simulink model "drive"  (R2024b)
settings: Solver=VariableStepAuto  StartTime=0.0  StopTime=10.0  RelTol=1e-3
InitFcn:
  | driveIni
values from neighbouring files (symbols this model uses):
  Par = problMatrices(Par)    [driveIni.m]
  psiR0 = [0.91; 0]    [driveIni.m]
  psiS0 = [1; 0]    [driveIni.m]
settings Model: Creator=PetrosK  LastModifiedBy=horak
settings DebuggingCC: UnderspecifiedInitializationDetection=Classic  MergeDetectMultiDrivingBlocksExec=none
settings ModelReferenceCC: PropagateSignalLabelsOutOfModel=off

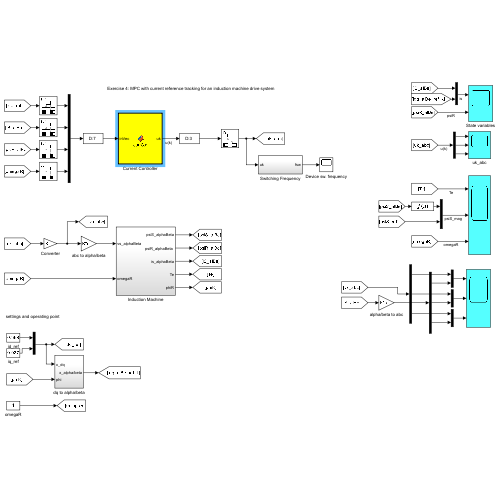
[thumbnail: Simulink's stored preview of the top-level diagram]
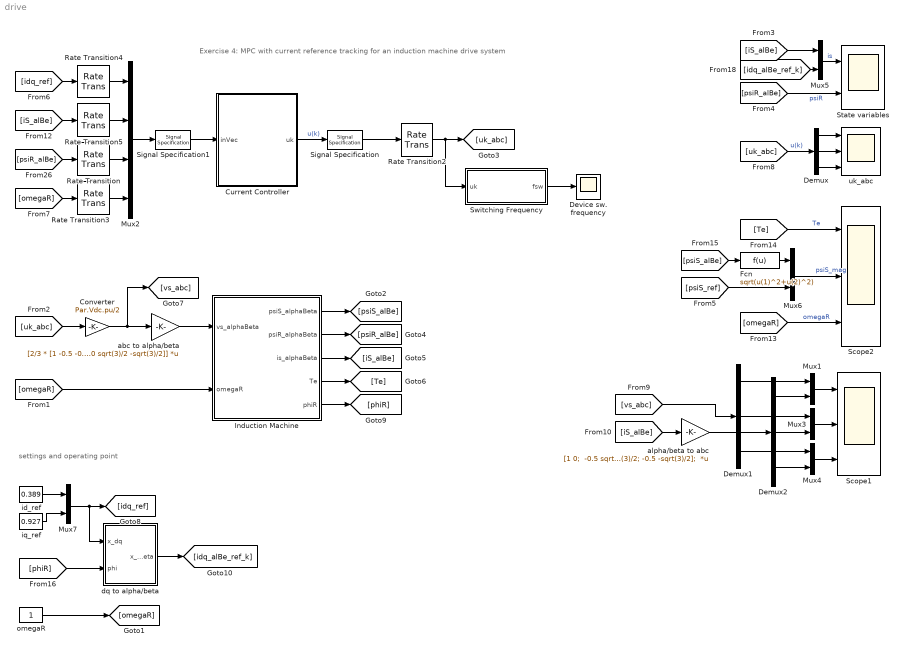
== system drive ==
  note: settings and operating point
  note: Exercise 4: MPC with current reference tracking for an induction machine drive system
  Converter : Gain  Gain=Par.Vdc.pu/2  SaturateOnIntegerOverflow=on  OutDataTypeStr=Inherit: Same as input  ParamDataTypeStr=Inherit: Same as input
  Current Controller : MATLAB Function  TreatAsAtomicUnit=on
  Demux : Demux  Outputs=3
  Demux1 : Demux  Outputs=3
  Demux2 : Demux  Outputs=3
  Device sw. frequency : Scope
  Fcn : Fcn  Expr=sqrt(u(1)^2+u(2)^2)
  Induction Machine : Subsystem
  Mux{1,3..7} (6 alike) : Mux  Inputs=2
  Mux2 : Mux
  Rate Transition{,3..5} (4 alike) : RateTransition  Deterministic=off  OutPortSampleTime=Par.Ts.control
  Rate Transition2 : RateTransition  OutPortSampleTime=Par.Ts.system
  Scope1 : Scope  NumInputPorts=3
  Scope2 : Scope  NumInputPorts=3
  Signal Specification : SignalSpecification  Dimensions=3
  Signal Specification1 : SignalSpecification  Dimensions=7
  State variables : Scope  NumInputPorts=2
  Switching Frequency : Subsystem
  abc to alpha/beta : Gain  Gain=[2/3 * [1 -0.5 -0.5;0 sqrt(3)/2 -sqrt(3)/2]]  Multiplication=Matrix(K*u)  SaturateOnIntegerOverflow=on  OutDataTypeStr=Inherit: Same as input  ParamDataTypeStr=Inherit: Same as input
  alpha/beta to abc : Gain  Gain="[1 0;  -0.5 sqrt(3)/2; -0.5 -sqrt(3)/2];"  Multiplication=Matrix(K*u)  SaturateOnIntegerOverflow=on  OutDataTypeStr=Inherit: Same as input  ParamDataTypeStr=Inherit: Same as input
  dq to alpha/beta : Subsystem
  id_ref : Constant  Value=0.389
  iq_ref : Constant  Value=0.927
  omegaR : Constant
  uk_abc : Scope  NumInputPorts=3
  wires:
  abc to alpha/beta/1 -> Induction Machine/1(vs_alphaBeta)
  [omegaR] -> Induction Machine/2(omegaR)
  [psiR_alBe] -> Rate Transition/1
  Current Controller/1(uk) -> Signal Specification/1  "u(k)"
  [omegaR] -> Rate Transition3/1
  Mux2/1 -> Signal Specification1/1
  Rate Transition3/1 -> Mux2/4
  Rate Transition/1 -> Mux2/3
  Signal Specification/1 -> Rate Transition2/1
  Rate Transition2/1 -> Switching Frequency/1(uk), [uk_abc]
  Signal Specification1/1 -> Current Controller/1(inVec)
  [uk_abc] -> Converter/1
  Converter/1 -> [vs_abc], abc to alpha/beta/1
  [psiR_alBe] -> State variables/2  "psiR"
  [uk_abc] -> Demux/1  "u(k)"
  Demux/1 -> uk_abc/1
  Demux/2 -> uk_abc/2
  Demux/3 -> uk_abc/3
  Induction Machine/1(psiS_alphaBeta) -> [psiS_alBe]
  Induction Machine/2("psiR_alphaBeta ") -> [psiR_alBe]
  Induction Machine/3(is_alphaBeta) -> [iS_alBe]
  Induction Machine/4(Te) -> [Te]
  Mux1/1 -> Scope1/1
  Mux3/1 -> Scope1/2
  Mux4/1 -> Scope1/3
  Demux1/1 -> Mux1/1
  alpha/beta to abc/1 -> Demux2/1
  Demux2/1 -> Mux1/2
  [iS_alBe] -> alpha/beta to abc/1
  Demux1/2 -> Mux3/1
  Demux1/3 -> Mux4/1
  Demux2/2 -> Mux3/2
  Demux2/3 -> Mux4/2
  [vs_abc] -> Demux1/1
  [omegaR] -> Scope2/3  "omegaR"
  Mux6/1 -> Scope2/2  "psiS_mag"
  [psiS_alBe] -> Fcn/1
  Rate Transition5/1 -> Mux2/2
  Rate Transition4/1 -> Mux2/1
  Fcn/1 -> Mux6/1
  [psiS_ref] -> Mux6/2
  omegaR/1 -> [omegaR]
  Switching Frequency/1(fsw) -> Device sw. frequency/1
  [idq_ref] -> Rate Transition4/1
  [iS_alBe] -> Rate Transition5/1
  [Te] -> Scope2/1  "Te"
  Mux7/1 -> dq to alpha/beta/1(x_dq), [idq_ref]
  [phiR] -> dq to alpha/beta/2(phi)
  Induction Machine/5(phiR) -> [phiR]
  dq to alpha/beta/1(x_alpha/beta) -> [idq_alBe_ref_k]
  Mux5/1 -> State variables/1  "is"
  [iS_alBe] -> Mux5/1
  [idq_alBe_ref_k] -> Mux5/2
  id_ref/1 -> Mux7/1
  iq_ref/1 -> Mux7/2

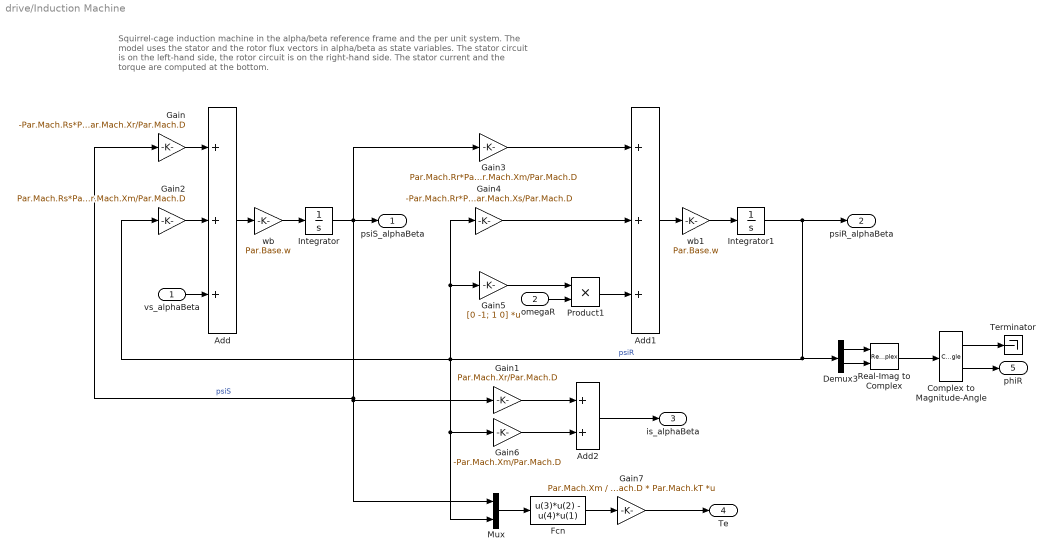
== system drive/Induction Machine ==
  note: Squirrel-cage induction machine in the alpha/beta reference frame and the per unit system.
      | The model uses the stator and the rotor flux vectors in alpha/beta as state variables.
      | The stator circuit is on the left-hand side, the rotor circuit is on the right-hand side.
      | The stator current and the torque are computed at the bottom.
  vs_alphaBeta : Inport
  omegaR : Inport  Port=2
  Add : Sum  Inputs=+++
  Add1 : Sum  Inputs=+++
  Add2 : Sum
  Complex to Magnitude-Angle : ComplexToMagnitudeAngle
  Demux3 : Demux  Outputs=2
  Fcn : Fcn  Expr=u(3)*u(2) - u(4)*u(1)
  Gain : Gain  Gain=-Par.Mach.Rs*Par.Mach.Xr/Par.Mach.D
  Gain1 : Gain  Gain=Par.Mach.Xr/Par.Mach.D
  Gain2 : Gain  Gain=Par.Mach.Rs*Par.Mach.Xm/Par.Mach.D
  Gain3 : Gain  Gain=Par.Mach.Rr*Par.Mach.Xm/Par.Mach.D
  Gain4 : Gain  Gain=-Par.Mach.Rr*Par.Mach.Xs/Par.Mach.D
  Gain5 : Gain  Gain=[0 -1; 1 0]  Multiplication=Matrix(K*u)
  Gain6 : Gain  Gain=-Par.Mach.Xm/Par.Mach.D
  Gain7 : Gain  Gain=Par.Mach.Xm / Par.Mach.D * Par.Mach.kT  Multiplication=Matrix(K*u)
  Integrator : Integrator  InitialCondition=psiS0
  Integrator1 : Integrator  InitialCondition=psiR0
  Mux : Mux  Inputs=2
  Product1 : Product
  Real-Imag to Complex : RealImagToComplex
  Terminator : Terminator
  wb : Gain  Gain=Par.Base.w
  wb1 : Gain  Gain=Par.Base.w
  psiS_alphaBeta : Outport
  "psiR_alphaBeta " : Outport  Port=2
  is_alphaBeta : Outport  Port=3
  Te : Outport  Port=4
  phiR : Outport  Port=5
  wires:
  vs_alphaBeta/1 -> Add/3
  Gain/1 -> Add/1
  Add/1 -> wb/1
  Gain3/1 -> Add1/1
  Add1/1 -> wb1/1
  Gain4/1 -> Add1/2
  Product1/1 -> Add1/3
  Gain2/1 -> Add/2
  Integrator/1 -> Gain3/1, psiS_alphaBeta/1, Mux/1, Gain1/1, Gain/1  "psiS"
  Integrator1/1 -> Demux3/1, Gain2/1, Mux/2, Gain6/1, Gain4/1, Gain5/1, "psiR_alphaBeta "/1  "psiR"
  Gain1/1 -> Add2/1
  Gain6/1 -> Add2/2
  Add2/1 -> is_alphaBeta/1
  Fcn/1 -> Gain7/1
  Gain7/1 -> Te/1
  Gain5/1 -> Product1/1
  omegaR/1 -> Product1/2
  Mux/1 -> Fcn/1
  wb1/1 -> Integrator1/1
  wb/1 -> Integrator/1
  Demux3/1 -> Real-Imag to Complex/1
  Demux3/2 -> Real-Imag to Complex/2
  Real-Imag to Complex/1 -> Complex to Magnitude-Angle/1
  Complex to Magnitude-Angle/2 -> phiR/1
  Complex to Magnitude-Angle/1 -> Terminator/1

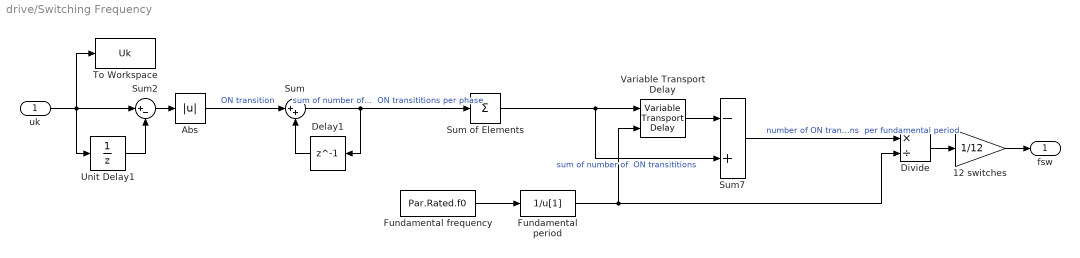
== system drive/Switching Frequency ==
  uk : Inport
  12 switches : Gain  Gain=1/12
  Abs : Abs  SaturateOnIntegerOverflow=off
  Delay1 : Delay  DelayLength=1  InitialCondition=0
  Divide : Product  Inputs=*/
  Fundamental frequency : Constant  Value=Par.Rated.f0
  Fundamental period : Fcn  Expr=1/u[1]
  Sum : Sum  Inputs=|++
  Sum of Elements : Sum  Inputs=+
  Sum2 : Sum  Inputs=|+-
  Sum7 : Sum  Inputs=-+  InputSameDT=on  SaturateOnIntegerOverflow=on  OutDataTypeStr=Inherit: Same as first input
  To Workspace : ToWorkspace  VariableName=Uk  SaveFormat=Structure With Time  SampleTime=-1
  Unit Delay1 : UnitDelay  SampleTime=-1  HasFrameUpgradeWarning=on
  Variable Transport Delay : VariableTransportDelay  VariableDelayType=Variable transport delay  MaximumDelay=0.05  MaximumPoints=2048*4  PadeOrder=2
  fsw : Outport
  wires:
  Sum/1 -> Sum of Elements/1, Delay1/1  "sum of number of  ON transititions per phase"
  Variable Transport Delay/1 -> Sum7/1
  Delay1/1 -> Sum/2
  Fundamental frequency/1 -> Fundamental period/1
  Fundamental period/1 -> Divide/2, Variable Transport Delay/2
  Sum7/1 -> Divide/1  "number of ON transitions  per fundamental period"
  uk/1 -> To Workspace/1, Sum2/1, Unit Delay1/1
  Unit Delay1/1 -> Sum2/2
  Sum2/1 -> Abs/1
  Abs/1 -> Sum/1  "ON transition"
  Divide/1 -> 12 switches/1
  12 switches/1 -> fsw/1
  Sum of Elements/1 -> Variable Transport Delay/1, Sum7/2  "sum of number of  ON transititions"

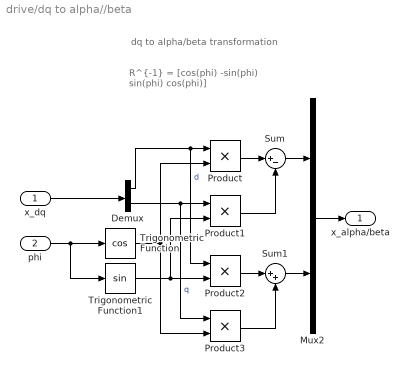
== system drive/dq to alpha//beta ==
  note: R^{-1} = [cos(phi) -sin(phi)
      |               sin(phi)  cos(phi)]
  note: dq to alpha/beta transformation
  x_dq : Inport
  phi : Inport  Port=2
  Demux : Demux  Outputs=2
  Mux2 : Mux  Inputs=2
  Product{,1..3} (4 alike) : Product  RndMeth=Zero
  Sum : Sum  Inputs=|+-
  Sum1 : Sum  Inputs=|++
  Trigonometric Function : Trigonometry  Operator=cos
  Trigonometric Function1 : Trigonometry
  x_alpha/beta : Outport
  wires:
  x_dq/1 -> Demux/1
  phi/1 -> Trigonometric Function/1, Trigonometric Function1/1
  Demux/1 -> Product/1, Product2/1  "d"
  Product/1 -> Sum/1
  Product1/1 -> Sum/2
  Sum/1 -> Mux2/1
  Demux/2 -> Product1/1, Product3/1  "q"
  Product2/1 -> Sum1/1
  Product3/1 -> Sum1/2
  Sum1/1 -> Mux2/2
  Mux2/1 -> x_alpha/beta/1
  Trigonometric Function1/1 -> Product2/2, Product1/2
  Trigonometric Function/1 -> Product/2, Product3/2

== matlab function drive/Current Controller ==
  data: inVec input; uk output size=[3,1]; Par parameter
function uk = currCtrl(inVec, Par)

% MPC with current reference tracking for an induction motor drive 
% system with prediction horizons exceeding one step
%
% Model Predictive Control of Power Electronic Systems, TAU, Tampere
% Petros Karamanakos, September 2025

% tell codegen that sphDec_solution is a MATLAB-only function and should not be compiled
coder.extrinsic('sphDec');

persistent Ukm1

% interface
idq_ref = inVec(1:2);       % stator current reference in dq (assumed to be constant over the prediction interval)
iAlphaBeta_k = inVec(3:4);	% stator current measurement in alpha/beta at time step k
psiR_alphaBeta_k = inVec(5:6); % rotor flux estimate in alpha/beta at time step k 
omegaR = inVec(7);          % rotor angular speed [pu]

% rotor flux angle at time step k
psiR_complex_k = psiR_alphaBeta_k(1) + 1i*psiR_alphaBeta_k(2);
phiR_k = angle(psiR_complex_k);

% parameters
Np = Par.Ctr.Np;        % prediction horizon (number of time steps)
dPhi = Par.Ts.control*Par.Base.w*omegaR;    % angle [rad] corresponding to one control sampling interval

% previous sequence of optimal switch positions
if isempty(Ukm1)
    Ukm1 = zeros(3*Np,1);
end
u_km1 = Ukm1(1:3);      % three-phase switch position applied at the previous time step k-1

%% current reference trajectory

% trajectory of the angular position of the dq reference frame 
% at time steps 1, 2, ... Np
PhiR = phiR_k + dPhi*[1:Np];

% stator current reference trajectory in alpha/beta 
% at time steps 1, 2, ... Np
Yref = [ cos(PhiR); sin(PhiR)]*idq_ref(1) ...
     + [-sin(PhiR); cos(PhiR)]*idq_ref(2);
Yref = Yref(:);     % vector
           
%% preparation of sphere decoding

% state vector at time step k
xk = [iAlphaBeta_k; psiR_alphaBeta_k];  

% load the problem matrices
Gamma = Par.Prob.Gamma;
Ypsilon = Par.Prob.Ypsilon;
Qtilde = Par.Prob.Qtilde;
E = Par.Prob.E;
S = Par.Prob.S;
Hinv = Par.Prob.Hinv;
V = Par.Prob.V;

% Theta matrix
Theta_a = -(Yref-Gamma*xk)'*Qtilde*Ypsilon;     % (5.13b)
Theta_b = -Par.Ctr.lambda*(E*u_km1)'*S;        	% (5.13b)
Theta = (Theta_a + Theta_b)';                   % 3Np x 1, (5.13b)

% unconstrained solution for Uk over k,...,k+Np-1
Uk_unc = -Hinv*Theta;  
Ubar_unc = V* Uk_unc ;      % unconstrained solution in V-space
                            
% educated guess: previous optimal switching sequence shifted in time
Uk_ini = zeros(3*Np,1); % trivial initial solution
Ubar_ini = V * Uk_ini;      % educated guess in V-space

% upper bound on the squared distance
rho = norm(Ubar_unc-Ubar_ini,2)^2;    % we use the *squared* distance / 2-norm here
rho = rho * (1+1e-9);       % we do this to avoid numerical problems and not finding any solution

%% solve sphere decoding problem

Uk_num = zeros(3*Np,1);  % numeric placeholder
searchFlag_num = 0;      % numeric placeholder

% call the sphere decoding algorithm
[~, Uk_tmp, ~, searchFlag_tmp] = sphDec(Uk_ini, [], 0, 1, 3*Np, rho, Ubar_unc, V, 0, u_km1);

% convert to numeric
Uk_num = double(Uk_tmp);
searchFlag_num = double(searchFlag_tmp);

% use numeric versions for all further code
Uk = Uk_num;
searchFlag = searchFlag_num;

if searchFlag == 0
    error('Sphere decoder did not find a solution'); 
else
    % *** uncomment this line to observe how many candidate switching
    % sequences are explored ***
    fprintf('The sphere decoder required %d iterations\n', int32(searchFlag));
end

%% output interface

Ukm1(1:3*Np) = Uk;
uk = Uk(1:3);

return
